simulink model "psbfftdemo"  (Simulink 6.0)
settings: Solver=ode45  StartTime=0.0  StopTime=1  RelTol=1e-3
libraries: simulink x1
settings Model: Creator=sybille  LastModifiedBy=batserve  ExtModeAutoUpdateStatusClock=off
settings DataIOCC: SignalLoggingName=sigsOut
settings OptimizationCC: BooleanDataType=off
settings DebuggingCC: CheckExecutionContextPreStartOutputMsg=on  CheckExecutionContextRuntimeOutputMsg=on  SolverPrmCheckMsg=none
settings HardwareCC: TargetUnknown=on

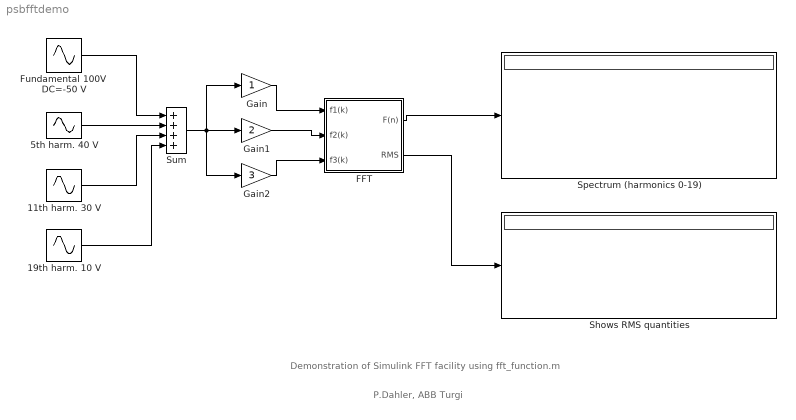
== system psbfftdemo ==
  note: Demonstration of Simulink FFT facility using fft_function.m
  note: P.Dahler, ABB Turgi
  "11th harm. 30 V " : Sin  Amplitude=30  Frequency=11*50*2*pi  SampleTime=0
  "19th harm. 10 V " : Sin  Amplitude=10  Frequency=19*50*2*pi  SampleTime=0
  "5th harm. 40 V " : Sin  Amplitude=40  Frequency=5*50*2*pi  SampleTime=0
  FFT : Subsystem  mask(Fast Fourier by Matlab Function){f1=50, Ts=500e-6, TsFFT=0.1, base=[1 1  1], nDec=0, mask=[1 -1 1], figure_N=1}
      mask prompts: f1 "Fundamental frequency f1 (Hz):"; Ts "Sampling time Ts (s):"; TsFFT "FFT Sampling time F(n)"; base "Base peak value (1 for absolute , size=[1 nSignals ])"; nDec "Decimals to display RMS values on spectrum (0 for no text)"; mask "Mask (nomally ones(1,nSignals))"; figure_N "Figure number"
      mask help:
      | This block  implements on-line FFT analysis  of 3  signals.
      |
      | It can be used as a "real time" analyzer during simulation (note speed reduction !) or off line by reading the signals from workspace after simulation.
      |
      | The F(n) output is a [N,3] matrix of the 3 signal spectra  (harmonic orders 0 to N-1), where N is the number of harmonics computed  given by : N= 1/f1/Ts/2.
      | The RMS output is a [5,3] matrix of 5 different RMS values of the 3 signals: Line 1=  Total RMS; 2=DC component; 3=RMS value of fundamental; 4= RMS value of harmonics; 6=Total  AC rms .
      |
      | The 3 spectra are displayed on specified Figure number. By selecting different Figure numbers multiple blocks can be used. A mask parameter can be used to modify plot appearance (1 or -1 row vector)
      |
      | See power_fftdemo model.
      mask init:
      | Navg=fix((1/f1)/Ts);
      mask Display: color('blue');disp('FFT')
  Fundamental 100V  DC=-50 V : Sin  Amplitude=100  Bias=-50  Frequency=50*2*pi  Phase=pi/2  SampleTime=0
  Gain : Gain  SaturateOnIntegerOverflow=on
  Gain1 : Gain  Gain=2  SaturateOnIntegerOverflow=on
  Gain2 : Gain  Gain=3  SaturateOnIntegerOverflow=on
  Shows RMS quantities : Display
      settings: Format=bank
  Spectrum (harmonics 0-19) : Display
      settings: Format=bank
  Sum : Sum  Inputs=++++  SaturateOnIntegerOverflow=on  InputSameDT=on
  wires:
  Fundamental 100V  DC=-50 V/1 -> Sum/1
  "5th harm. 40 V "/1 -> Sum/2
  "11th harm. 30 V "/1 -> Sum/3
  FFT/2(RMS) -> Shows RMS quantities/1
  FFT/1(F(n)) -> Spectrum (harmonics 0-19)/1
  Gain/1 -> FFT/1(f1(k))
  Gain1/1 -> FFT/2(f2(k))
  Gain2/1 -> FFT/3(f3(k))
  Sum/1 -> Gain1/1, Gain/1, Gain2/1
  "19th harm. 10 V "/1 -> Sum/4

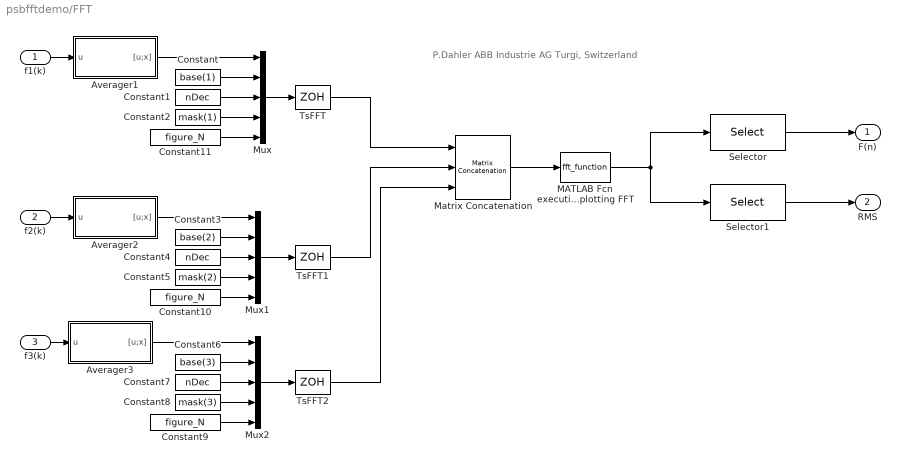
== system psbfftdemo/FFT ==
  note: P.Dahler
      | ABB Industrie AG
      | Turgi, Switzerland
  f1(k) : Inport  Port=1  LatchInput=off
  f2(k) : Inport  Port=2  LatchInput=off
  f3(k) : Inport  Port=3  LatchInput=off
  Averager1 : Subsystem  mask(Shift Register with discrete state space block){Navg=Navg, x0=0, Ts=Ts}
      mask prompts: Navg "Number of Samples inl. in(k)"; x0 "Inititial Condition"; Ts "Sample Time (-1 for inherited)"
      mask help: This block is a shift register storing values [u(k) u(k-1) ... u(k-(Navg-1))]' . This vector can be used for a FFT analysis.
      mask init:
      | %Discrete State Space model of averager
      | %one scalar input
      | %Navg sized output [in(k) in(k-1) .... in(k-(Navg-1))]
      | Q=eye(Navg-1);
      | A=[Q(:,2:length(Q))  Q(:,1)] ;
      | A(1,Navg-1)=0;
      | B=[1 ; zeros(Navg-2,1)];
      | C=eye(Navg) ;
      | C=C(:,2:length(C));
      | D=[1 ; zeros(Navg-1,1)];
      mask Help: This block is a shift register storing values [u(k) u(k-1) ... u(k-(Navg-1))]' . This vector can be used for a FFT analysis.
      mask Display: disp('Shift\nRegister')
  Averager2 : Subsystem  mask(Shift Register with discrete state space block){Navg=Navg, x0=0, Ts=Ts}
      mask prompts: Navg "Number of Samples inl. in(k)"; x0 "Inititial Condition"; Ts "Sample Time (-1 for inherited)"
      mask help: This block is a shift register storing values [u(k) u(k-1) ... u(k-(Navg-1))]' . This vector can be used for a FFT analysis.
      mask init: same as psbfftdemo/FFT/Averager1
      mask Help: This block is a shift register storing values [u(k) u(k-1) ... u(k-(Navg-1))]' . This vector can be used for a FFT analysis.
      mask Display: disp('Shift\nRegister')
  Averager3 : Subsystem  mask(Shift Register with discrete state space block){Navg=Navg, x0=0, Ts=Ts}
      mask prompts: Navg "Number of Samples inl. in(k)"; x0 "Inititial Condition"; Ts "Sample Time (-1 for inherited)"
      mask help: This block is a shift register storing values [u(k) u(k-1) ... u(k-(Navg-1))]' . This vector can be used for a FFT analysis.
      mask init: same as psbfftdemo/FFT/Averager1
      mask Help: This block is a shift register storing values [u(k) u(k-1) ... u(k-(Navg-1))]' . This vector can be used for a FFT analysis.
      mask Display: disp('Shift\nRegister')
  Constant : Constant  Value=base(1)
  Constant1 : Constant  Value=nDec
  Constant10 : Constant  Value=figure_N
  Constant11 : Constant  Value=figure_N
  Constant2 : Constant  Value=mask(1)
  Constant3 : Constant  Value=base(2)
  Constant4 : Constant  Value=nDec
  Constant5 : Constant  Value=mask(2)
  Constant6 : Constant  Value=base(3)
  Constant7 : Constant  Value=nDec
  Constant8 : Constant  Value=mask(3)
  Constant9 : Constant  Value=figure_N
  MATLAB Fcn executing and plotting FFT : MATLABFcn  MATLABFcn=fft_function  OutputDimensions="[ceil(Navg/2) + 5  3]"  Output1D=off
  Matrix Concatenation : simulink/Math Operations/Matrix Concatenation  numInports=3  catMethod=Horizontal
  Mux : Mux  Inputs=5
  Mux1 : Mux  Inputs=5
  Mux2 : Mux  Inputs=5
  Selector : Selector  InputType=Matrix  Elements=[1:ceil(Navg/2)]  Rows=1:ceil(Navg/2)  Columns=1:3  InputPortWidth=ceil(Navg/2) + 5
  Selector1 : Selector  InputType=Matrix  Elements=[1:ceil(Navg/2)]  Rows=ceil(Navg/2)+1 : ceil(Navg/2)+5  Columns=1:3  InputPortWidth=ceil(Navg/2) + 5
  TsFFT : ZeroOrderHold  SampleTime=TsFFT
  TsFFT1 : ZeroOrderHold  SampleTime=TsFFT
  TsFFT2 : ZeroOrderHold  SampleTime=TsFFT
  F(n) : Outport
  RMS : Outport  Port=2
  wires:
  Matrix Concatenation/1 -> MATLAB Fcn executing and plotting FFT/1
  TsFFT2/1 -> Matrix Concatenation/3
  Constant6/1 -> Mux2/2
  Constant7/1 -> Mux2/3
  f3(k)/1 -> Averager3/1(u)
  Mux2/1 -> TsFFT2/1
  Averager3/1("[u;x]") -> Mux2/1
  Constant8/1 -> Mux2/4
  TsFFT1/1 -> Matrix Concatenation/2
  TsFFT/1 -> Matrix Concatenation/1
  Constant3/1 -> Mux1/2
  Constant4/1 -> Mux1/3
  f2(k)/1 -> Averager2/1(u)
  Mux1/1 -> TsFFT1/1
  Averager2/1("[u;x]") -> Mux1/1
  Constant5/1 -> Mux1/4
  MATLAB Fcn executing and plotting FFT/1 -> Selector1/1, Selector/1
  Selector/1 -> F(n)/1
  Selector1/1 -> RMS/1
  Constant/1 -> Mux/2
  Constant1/1 -> Mux/3
  f1(k)/1 -> Averager1/1(u)
  Mux/1 -> TsFFT/1
  Averager1/1("[u;x]") -> Mux/1
  Constant2/1 -> Mux/4
  Constant9/1 -> Mux2/5
  Constant10/1 -> Mux1/5
  Constant11/1 -> Mux/5

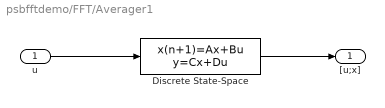
== system psbfftdemo/FFT/Averager1 ==
  u : Inport  Port=1  LatchInput=off
  Discrete State-Space : DiscreteStateSpace  A=A  B=B  C=C  D=D  X0=x0  SampleTime=Ts
  "[u;x]" : Outport
  wires:
  Discrete State-Space/1 -> "[u;x]"/1
  u/1 -> Discrete State-Space/1

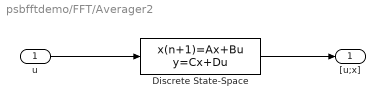
== system psbfftdemo/FFT/Averager2 ==
  u : Inport  Port=1  LatchInput=off
  Discrete State-Space : DiscreteStateSpace  A=A  B=B  C=C  D=D  X0=x0  SampleTime=Ts
  "[u;x]" : Outport
  wires:
  u/1 -> Discrete State-Space/1
  Discrete State-Space/1 -> "[u;x]"/1

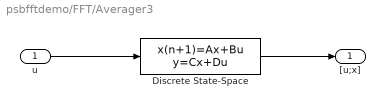
== system psbfftdemo/FFT/Averager3 ==
  u : Inport  Port=1  LatchInput=off
  Discrete State-Space : DiscreteStateSpace  A=A  B=B  C=C  D=D  X0=x0  SampleTime=Ts
  "[u;x]" : Outport
  wires:
  Discrete State-Space/1 -> "[u;x]"/1
  u/1 -> Discrete State-Space/1
